simulink model "schema_simulink"  (R2014a)
settings: Solver=ode45  StartTime=0.0  StopTime=2  RelTol=1e-3
libraries: cstblocks x3, simulink x1
settings Model: Creator=User  LastModifiedBy=User

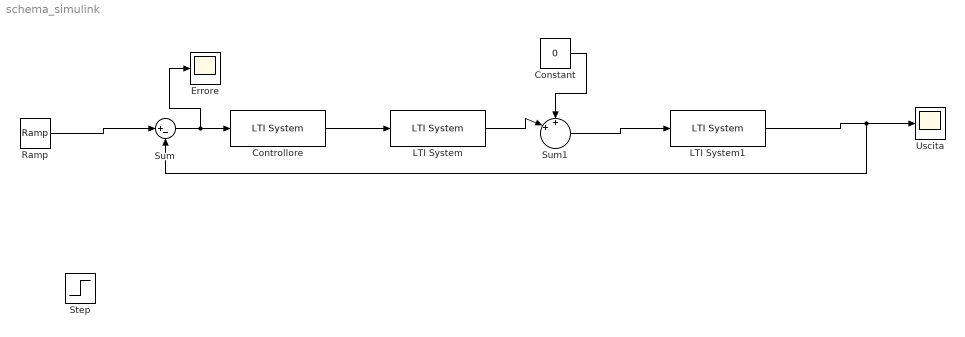
== system schema_simulink ==
  Constant : Constant  Value=0
  Controllore : cstblocks/LTI System  sys=C  IC=[]
  "Errore " : Scope
  LTI System : cstblocks/LTI System  sys=F1  IC=[]
  LTI System1 : cstblocks/LTI System  sys=F2  IC=[]
  Ramp : simulink/Sources/Ramp  slope=1  start=0  X0=0
  Step : Step  Time=0  After=0  SampleTime=0
  Sum : Sum  Inputs=|+-
  Sum1 : Sum  Inputs=++||
  "Uscita " : Scope
  wires:
  Sum/1 -> "Errore "/1, Controllore/1
  Controllore/1 -> LTI System/1
  LTI System/1 -> Sum1/2
  Constant/1 -> Sum1/1
  Sum1/1 -> LTI System1/1
  LTI System1/1 -> Sum/2, "Uscita "/1
  Ramp/1 -> Sum/1
